simulink model "twolevelwithconstantdcvoltage_tuned_2017"  (R2017b)
settings: Solver=FixedStepAuto  StartTime=0.0  StopTime=30  FixedStep=Ts  MaxStep=1e-4  RelTol=1e-3  EnableMultiTasking=on
undefined symbols (not defined in the file): Ts
libraries: powerlib x18, powerlib_meascontrol x10, simulink x3
settings Model: Creator=Eren  LastModifiedBy=Eren
settings DataIOCC: LimitDataPoints=on
settings OptimizationCC: LifeSpan=inf
settings DebuggingCC: AllowSymbolicDim=off  SFUnexpectedBacktrackingDiag=warning  SFNoUnconditionalDefaultTransitionDiag=warning  SFExecutionAtInitializationDiag=none
settings ModelReferenceCC: PropagateSignalLabelsOutOfModel=off
settings CodeAppCC: StateflowObjectComments=on
settings GRTTargetCC: TargetLangStandard=C89/C90 (ANSI)
settings ConfigComp: CovMetricSettings=dw  CovHtmlReporting=on  CovSaveCumulativeToWorkspaceVar=on  CovSaveSingleToWorkspaceVar=on  CovExternalEMLEnable=off
settings SimscapeCC: SimscapeNormalizeSystem=off

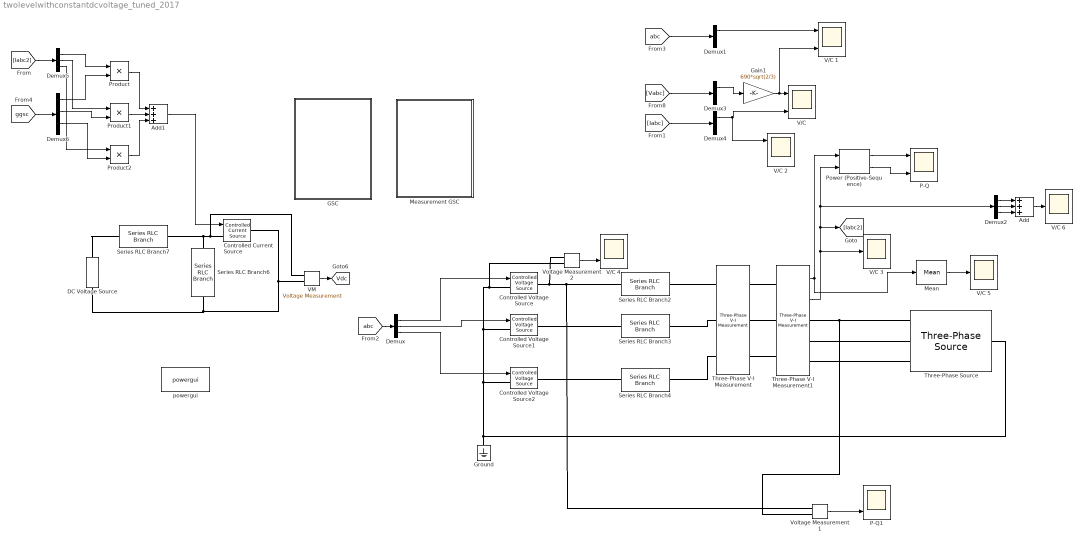
== system twolevelwithconstantdcvoltage_tuned_2017 ==
  Add : Sum  Inputs=3
  Add1 : Sum  Inputs=3
  Controlled Current Source : powerlib/Electrical Sources/Controlled Current Source  Initialize=off  Source_Type=AC  Amplitude=0  Phase=0  Frequency=0  Measurements=None
  Controlled Voltage Source : powerlib/Electrical Sources/Controlled Voltage Source  Initialize=off  Source_Type=AC  Amplitude=0  Phase=0  Frequency=0  Measurements=None
  Controlled Voltage Source1 : powerlib/Electrical Sources/Controlled Voltage Source  Initialize=on  Source_Type=AC  Amplitude=0  Phase=0  Frequency=0  Measurements=None
  Controlled Voltage Source2 : powerlib/Electrical Sources/Controlled Voltage Source  Initialize=on  Source_Type=AC  Amplitude=0  Phase=0  Frequency=0  Measurements=None
  DC Voltage Source : powerlib/Electrical Sources/DC Voltage Source  Amplitude=1300  Measurements=None
  Demux{,1..5} (6 alike) : Demux  Outputs=3
  Demux6 : Demux  Outputs=6
  GSC : Subsystem
  Gain1 : Gain  Gain=690*sqrt(2/3)
  Ground : powerlib/Elements/Ground  LConnTagsString=a
  Mean : powerlib_meascontrol/Measurements/Mean  Freq=50  Vinit=0  Ts=Ts
  Measurement GSC : Subsystem
  P-Q : Scope  NumInputPorts=2
  P-Q1 : Scope  NumInputPorts=2
  Power (Positive-Sequence) : powerlib_meascontrol/Measurements/Power (Positive-Sequence)  Freq=50  Vinit=[0, 0]  Iinit=[0, 0]  Ts=Ts
      settings: SourceProductName=Simscape Power Systems  SourceProductBaseCode=PS
  Product : Product
  Product1 : Product
  Product2 : Product
  Series RLC Branch2 : powerlib/Elements/Series RLC Branch  LConnTagsString=__new0  RConnTagsString=__new0  BranchType=L  Resistance=1  Inductance=2e-4  SetiL0=off  InitialCurrent=0  Capacitance=1e-6  Setx0=off  InitialVoltage=0  Measurements=None
  Series RLC Branch3 : powerlib/Elements/Series RLC Branch  LConnTagsString=__new0  RConnTagsString=__new0  BranchType=L  Resistance=1  Inductance=2e-4  SetiL0=off  InitialCurrent=0  Capacitance=1e-6  Setx0=off  InitialVoltage=0  Measurements=None
  Series RLC Branch4 : powerlib/Elements/Series RLC Branch  LConnTagsString=__new0  RConnTagsString=__new0  BranchType=L  Resistance=1  Inductance=2e-4  SetiL0=off  InitialCurrent=0  Capacitance=1e-6  Setx0=off  InitialVoltage=0  Measurements=None
  Series RLC Branch6 : powerlib/Elements/Series RLC Branch  LConnTagsString=__new0  RConnTagsString=__new0  BranchType=C  Resistance=1  Inductance=1e-4  SetiL0=off  InitialCurrent=0  Capacitance=27e-3  Setx0=off  InitialVoltage=0  Measurements=None
  Series RLC Branch7 : powerlib/Elements/Series RLC Branch  LConnTagsString=__new0  RConnTagsString=__new0  BranchType=R  Resistance=(120000)/(2.75*10^6)  Inductance=1e-3  SetiL0=off  InitialCurrent=0  Capacitance=1e-6  Setx0=off  InitialVoltage=0  Measurements=None
  Three-Phase V-I Measurement : powerlib/Measurements/Three-Phase V-I Measurement  VoltageMeasurement=phase-to-ground  SetLabelV=on  LabelV=Vabc  Vpu=on  VpuLL=off  CurrentMeasurement=yes  SetLabelI=on  LabelI=Iabc  Ipu=on  Pbase=2.75e6  Vbase=690  OutputType=Complex  PhasorSimulation=off  PSBequivalent=0
  Three-Phase V-I Measurement1 : powerlib/Measurements/Three-Phase V-I Measurement  VoltageMeasurement=phase-to-ground  SetLabelV=off  LabelV=Vabc  Vpu=off  VpuLL=off  CurrentMeasurement=yes  SetLabelI=off  LabelI=Iabc  Ipu=off  Pbase=2.75e6  Vbase=690  OutputType=Complex  PhasorSimulation=off  PSBequivalent=0
  Three-Phase Source : powerlib/Electrical Sources/Three-Phase Source  InternalConnection=Yn  VoltagePhases=off  Voltage=690  PhaseAngle=0  Voltage_phases=[25e3 25e3 25e3]/sqrt(3)  PhaseAngles_phases=[0 -120 +120]  Frequency=50  NonIdealSource=on  SpecifyImpedance=off  Resistance=3e-5  Inductance=1e-5  ShortCircuitLevel=500e6  BaseVoltage=690  XRratio=7  BusType=swing  Pref=10e3  Qref=0  Prefabc=[10e3, 10e3, 10e3]  Qrefabc=[0, 0, 0]  Qmin=-inf  Qmax=inf
  V/C {,1..2,4} (4 alike) : Scope  NumInputPorts=2
  V/C 3 : Scope
  V/C 5 : Scope
  V/C 6 : Scope
  VM : powerlib/Measurements/Voltage Measurement  PhasorSimulation=off  OutputType=Complex  PSBequivalent=0
  Voltage Measurement1 : powerlib/Measurements/Voltage Measurement  PhasorSimulation=off  OutputType=Complex  PSBequivalent=0
  Voltage Measurement2 : powerlib/Measurements/Voltage Measurement  PhasorSimulation=off  OutputType=Complex  PSBequivalent=0
  powergui : powerlib/powergui  Priority=1  SimulationMode=Continuous  SampleTime=50e-6  frequency=60  Iterations=50  frequencyindice=60  Pbase=100e6  ErrMax=1e-4  UnitsV=kV  UnitsW=MW  buscounter=0  FunctionMessages=off  echomessages=off  EnableUseOfTLC=off  CurrentSourceSwitches=off  DisableSnubberDevices=off  DisableRonSwitches=off  DisableVfSwitches=off  DisplayEquations=off  SolverType=Tustin/Backward Euler (TBE)  Interpol=off  ExternalGateDelay=off  methode=off  Ts=100  x0status=blocks  SPID=on  SwTol=0  HookPort=off  RestoreLinks=warning  ResistiveCurrentMeasurement=off  Frange=[0:2:500]  Ylog=off  Xlog=on  ShowGrid=off  save=off  variable=ZData  structure=0  ZoomFFT=off  StartTime=0.0  cycles=1  DisplayStyle=1  fundamental=60  FreqAxis=off  MaxFrequency=1000  frequencyindicesteady=1  RmsSteady=1  display=off
  tag scope: Vdc=global
  wires:
  Demux4/1 -> V/C 2/1, "V/C "/2
  Demux3/1 -> Gain1/1
  [Vabc] -> Demux3/1
  VM/1 -> [Vdc]
  Power (Positive-Sequence)/1 -> P-Q/1
  Power (Positive-Sequence)/2 -> P-Q/2
  [Iabc] -> Demux4/1
  Three-Phase V-I Measurement1/1 -> Power (Positive-Sequence)/1, Mean/1
  Three-Phase V-I Measurement1/2 -> V/C 3/1, [Iabc2], Power (Positive-Sequence)/2, Demux2/1
  [abc] -> Demux/1
  Demux/1 -> Controlled Voltage Source/1
  Demux/2 -> Controlled Voltage Source1/1
  Demux/3 -> Controlled Voltage Source2/1
  [abc] -> Demux1/1
  Demux1/1 -> V/C 1/1
  Gain1/1 -> V/C 1/2, "V/C "/1
  Voltage Measurement1/1 -> P-Q1/2
  Voltage Measurement2/1 -> V/C 4/2
  Mean/1 -> V/C 5/1
  Demux2/1 -> Add/1
  Demux2/2 -> Add/2
  Demux2/3 -> Add/3
  Add/1 -> V/C 6/1
  [Iabc2] -> Demux5/1
  [ggsc] -> Demux6/1
  Demux5/1 -> Product/1
  Demux6/1 -> Product/2
  Demux5/2 -> Product1/1
  Demux6/3 -> Product1/2
  Demux5/3 -> Product2/1
  Demux6/5 -> Product2/2
  Product/1 -> Add1/1
  Product1/1 -> Add1/2
  Product2/1 -> Add1/3
  Add1/1 -> Controlled Current Source/1
  connections:
  Three-Phase V-I Measurement1/RConn1 -- Three-Phase Source/RConn1 -- Voltage Measurement1/LConn2
  Series RLC Branch7/LConn1 -- DC Voltage Source/RConn1
  Series RLC Branch2/RConn1 -- Three-Phase V-I Measurement/LConn1
  Series RLC Branch6/RConn1 -- VM/LConn2 -- Controlled Current Source/RConn1 -- DC Voltage Source/LConn1
  Three-Phase V-I Measurement/RConn1 -- Three-Phase V-I Measurement1/LConn1
  Three-Phase V-I Measurement1/LConn2 -- Three-Phase V-I Measurement/RConn2
  Three-Phase V-I Measurement/RConn3 -- Three-Phase V-I Measurement1/LConn3
  Controlled Voltage Source/LConn1 -- Voltage Measurement2/LConn2 -- Ground/LConn1 -- Three-Phase Source/LConn1 -- Controlled Voltage Source2/LConn1 -- Controlled Voltage Source1/LConn1
  Series RLC Branch3/LConn1 -- Controlled Voltage Source1/RConn1
  Series RLC Branch4/RConn1 -- Three-Phase V-I Measurement/LConn3
  Series RLC Branch2/LConn1 -- Voltage Measurement1/LConn1 -- Voltage Measurement2/LConn1 -- Controlled Voltage Source/RConn1
  Series RLC Branch3/RConn1 -- Three-Phase V-I Measurement/LConn2
  Series RLC Branch4/LConn1 -- Controlled Voltage Source2/RConn1
  Three-Phase Source/RConn2 -- Three-Phase V-I Measurement1/RConn2
  Three-Phase Source/RConn3 -- Three-Phase V-I Measurement1/RConn3
  Series RLC Branch6/LConn1 -- VM/LConn1 -- Controlled Current Source/LConn1 -- Series RLC Branch7/RConn1

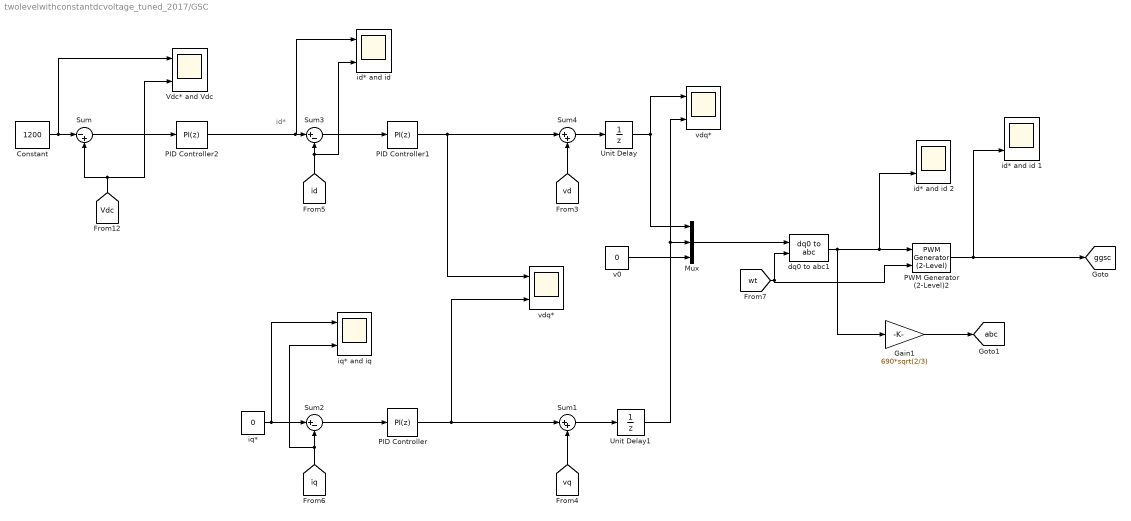
== system twolevelwithconstantdcvoltage_tuned_2017/GSC ==
  note: id*
  Constant : Constant  Value=1200
  Gain1 : Gain  Gain=690*sqrt(2/3)
  Mux : Mux  Inputs=3
  PID Controller : simulink/Continuous/PID Controller  Controller=PI  TimeDomain=Discrete-time  SampleTime=-1  IntegratorMethod=Forward Euler  FilterMethod=Forward Euler  Form=Parallel  UseFilter=on  ControllerParametersSource=internal  P=49.7840114924255  I=37375.3273073798  D=0  N=100  InitialConditionSource=internal  InitialConditionForIntegrator=0  InitialConditionForFilter=0  ExternalReset=none  LimitOutput=on  UpperSaturationLimit=2  LowerSaturationLimit=-2  LinearizeAsGain=on  AntiWindupMode=none  Kb=1  TrackingMode=off  Kt=1  PParamMin=[]  PParamMax=[]  IParamMin=[]  IParamMax=[]  DParamMin=[]  DParamMax=[]  NParamMin=[]  NParamMax=[]  KbParamMin=[]  KbParamMax=[]  KtParamMin=[]  KtParamMax=[]  POutMin=[]  POutMax=[]  IOutMin=[]  IOutMax=[]  DOutMin=[]  DOutMax=[]  NOutMin=[]  NOutMax=[]  KbOutMin=[]  KbOutMax=[]  KtOutMin=[]  KtOutMax=[]  IntegratorOutMin=[]  IntegratorOutMax=[]  FilterOutMin=[]  FilterOutMax=[]  SumOutMin=[]  SumOutMax=[]  SumI1OutMin=[]  SumI1OutMax=[]  SumI2OutMin=[]  SumI2OutMax=[]  SumI3OutMin=[]  SumI3OutMax=[]  SumDOutMin=[]  SumDOutMax=[]  SaturationOutMin=[]  SaturationOutMax=[]  IntegratorContinuousStateAttributes=''  IntegratorStateMustResolveToSignalObject=off  IntegratorRTWStateStorageClass=Auto  FilterContinuousStateAttributes=''  FilterStateMustResolveToSignalObject=off  FilterRTWStateStorageClass=Auto  DifferentiatorICPrevScaledInput=0  DifferentiatorOutMin=[]  DifferentiatorOutMax=[]  InitialConditionSetting=State (most efficient)  FilterDiffOutCoefMin=[]  FilterDiffOutCoefMax=[]  SumDenOutMin=[]  SumDenOutMax=[]  SumNumOutMin=[]  SumNumOutMax=[]  ReciprocalOutMin=[]  ReciprocalOutMax=[]  DivideOutMin=[]  DivideOutMax=[]  TunerSelectOption=Transfer Function Based (PID Tuner App)
  PID Controller1 : simulink/Continuous/PID Controller  Controller=PI  TimeDomain=Discrete-time  SampleTime=-1  IntegratorMethod=Forward Euler  FilterMethod=Forward Euler  Form=Parallel  UseFilter=on  ControllerParametersSource=internal  P=34.0158922210728  I=17493.3134828869  D=0  N=100  InitialConditionSource=internal  InitialConditionForIntegrator=0  InitialConditionForFilter=0  ExternalReset=none  LimitOutput=on  UpperSaturationLimit=1  LowerSaturationLimit=-1  LinearizeAsGain=on  AntiWindupMode=none  Kb=1  TrackingMode=off  Kt=1  PParamMin=[]  PParamMax=[]  IParamMin=[]  IParamMax=[]  DParamMin=[]  DParamMax=[]  NParamMin=[]  NParamMax=[]  KbParamMin=[]  KbParamMax=[]  KtParamMin=[]  KtParamMax=[]  POutMin=[]  POutMax=[]  IOutMin=[]  IOutMax=[]  DOutMin=[]  DOutMax=[]  NOutMin=[]  NOutMax=[]  KbOutMin=[]  KbOutMax=[]  KtOutMin=[]  KtOutMax=[]  IntegratorOutMin=[]  IntegratorOutMax=[]  FilterOutMin=[]  FilterOutMax=[]  SumOutMin=[]  SumOutMax=[]  SumI1OutMin=[]  SumI1OutMax=[]  SumI2OutMin=[]  SumI2OutMax=[]  SumI3OutMin=[]  SumI3OutMax=[]  SumDOutMin=[]  SumDOutMax=[]  SaturationOutMin=[]  SaturationOutMax=[]  IntegratorContinuousStateAttributes=''  IntegratorStateMustResolveToSignalObject=off  IntegratorRTWStateStorageClass=Auto  FilterContinuousStateAttributes=''  FilterStateMustResolveToSignalObject=off  FilterRTWStateStorageClass=Auto  DifferentiatorICPrevScaledInput=0  DifferentiatorOutMin=[]  DifferentiatorOutMax=[]  InitialConditionSetting=State (most efficient)  FilterDiffOutCoefMin=[]  FilterDiffOutCoefMax=[]  SumDenOutMin=[]  SumDenOutMax=[]  SumNumOutMin=[]  SumNumOutMax=[]  ReciprocalOutMin=[]  ReciprocalOutMax=[]  DivideOutMin=[]  DivideOutMax=[]  TunerSelectOption=Transfer Function Based (PID Tuner App)
  PID Controller2 : simulink/Continuous/PID Controller  Controller=PI  TimeDomain=Discrete-time  SampleTime=-1  IntegratorMethod=Forward Euler  FilterMethod=Forward Euler  Form=Parallel  UseFilter=on  ControllerParametersSource=internal  P=83655.09858372  I=42227.4588739829  D=0  N=100  InitialConditionSource=internal  InitialConditionForIntegrator=0  InitialConditionForFilter=0  ExternalReset=none  LimitOutput=off  UpperSaturationLimit=inf  LowerSaturationLimit=-inf  LinearizeAsGain=on  AntiWindupMode=none  Kb=1  TrackingMode=off  Kt=1  PParamMin=[]  PParamMax=[]  IParamMin=[]  IParamMax=[]  DParamMin=[]  DParamMax=[]  NParamMin=[]  NParamMax=[]  KbParamMin=[]  KbParamMax=[]  KtParamMin=[]  KtParamMax=[]  POutMin=[]  POutMax=[]  IOutMin=[]  IOutMax=[]  DOutMin=[]  DOutMax=[]  NOutMin=[]  NOutMax=[]  KbOutMin=[]  KbOutMax=[]  KtOutMin=[]  KtOutMax=[]  IntegratorOutMin=[]  IntegratorOutMax=[]  FilterOutMin=[]  FilterOutMax=[]  SumOutMin=[]  SumOutMax=[]  SumI1OutMin=[]  SumI1OutMax=[]  SumI2OutMin=[]  SumI2OutMax=[]  SumI3OutMin=[]  SumI3OutMax=[]  SumDOutMin=[]  SumDOutMax=[]  SaturationOutMin=[]  SaturationOutMax=[]  IntegratorContinuousStateAttributes=''  IntegratorStateMustResolveToSignalObject=off  IntegratorRTWStateStorageClass=Auto  FilterContinuousStateAttributes=''  FilterStateMustResolveToSignalObject=off  FilterRTWStateStorageClass=Auto  DifferentiatorICPrevScaledInput=0  DifferentiatorOutMin=[]  DifferentiatorOutMax=[]  InitialConditionSetting=State (most efficient)  FilterDiffOutCoefMin=[]  FilterDiffOutCoefMax=[]  SumDenOutMin=[]  SumDenOutMax=[]  SumNumOutMin=[]  SumNumOutMax=[]  ReciprocalOutMin=[]  ReciprocalOutMax=[]  DivideOutMin=[]  DivideOutMax=[]  TunerSelectOption=Transfer Function Based (PID Tuner App)
  PWM Generator (2-Level)2 : powerlib_meascontrol/Pulse & Signal Generators/PWM Generator (2-Level)  ModulatorType=Three-phase bridge (6 pulses)  ModulatorMode=Synchronized  Fc=50*60  Pc=90  nF=100  MinMax="[ -1  1 ]"  SamplingTechnique=Natural  ModulatingSignals=off  m=0.8  Freq=60  Phase=0  Ts=Ts  ShowCarrierOutport=off
      settings: SourceProductName=Simscape Power Systems
  Sum : Sum  Inputs=|-+
  Sum1 : Sum  Inputs=|++
  Sum2 : Sum  Inputs=|+-
  Sum3 : Sum  Inputs=|+-
  Sum4 : Sum  Inputs=|++
  Unit Delay : UnitDelay  SampleTime=Ts
  Unit Delay1 : UnitDelay  SampleTime=Ts
  Vdc* and Vdc : Scope  NumInputPorts=2
  dq0 to abc1 : powerlib_meascontrol/Transformations/dq0 to abc  Alignment=90 degrees behind phase A axis
  "id* and id " : Scope  NumInputPorts=2
  id* and id 1 : Scope  NumInputPorts=2
  id* and id 2 : Scope  NumInputPorts=2
  iq* : Constant  Value=0
  "iq* and iq " : Scope  NumInputPorts=2
  v0 : Constant  Value=0
  vdq* : Scope  NumInputPorts=2
  "vdq* " : Scope  NumInputPorts=2
  tag scope: abc=global, ggsc=global
  wires:
  PWM Generator (2-Level)2/1 -> id* and id 1/2, [ggsc]
  iq*/1 -> "iq* and iq "/1, Sum2/1
  Sum3/1 -> PID Controller1/1
  [iq] -> Sum2/2, "iq* and iq "/2
  PID Controller/1 -> Sum1/1, vdq*/2
  [vq] -> Sum1/2
  [id] -> "id* and id "/2, Sum3/2
  Sum2/1 -> PID Controller/1
  [vd] -> Sum4/2
  PID Controller1/1 -> Sum4/1, vdq*/1
  Sum4/1 -> Unit Delay/1
  Mux/1 -> dq0 to abc1/1
  [wt] -> dq0 to abc1/2, PWM Generator (2-Level)2/2
  Sum1/1 -> Unit Delay1/1
  v0/1 -> Mux/3
  [Vdc] -> Vdc* and Vdc/2, Sum/2
  Sum/1 -> PID Controller2/1
  Constant/1 -> Vdc* and Vdc/1, Sum/1
  PID Controller2/1 -> "id* and id "/1, Sum3/1
  dq0 to abc1/1 -> Gain1/1, id* and id 2/2, PWM Generator (2-Level)2/1
  Gain1/1 -> [abc]
  Unit Delay/1 -> Mux/1, "vdq* "/1
  Unit Delay1/1 -> "vdq* "/2, Mux/2

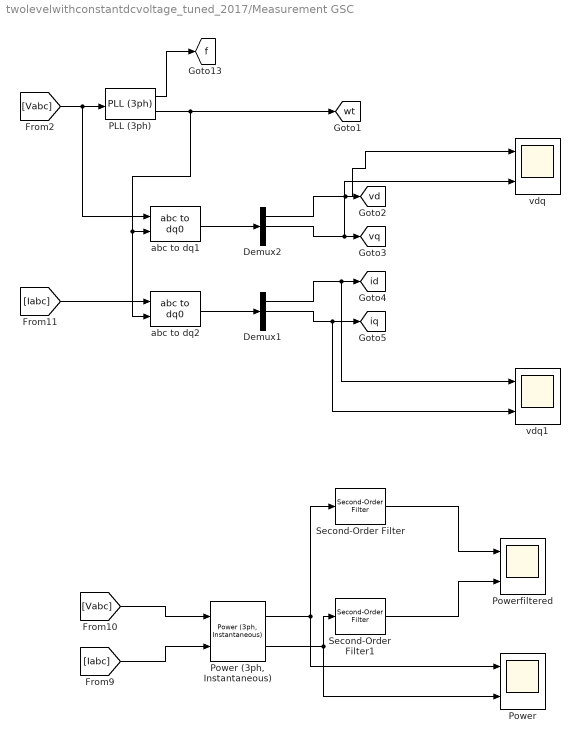
== system twolevelwithconstantdcvoltage_tuned_2017/Measurement GSC ==
  Demux1 : Demux  Outputs=3
  Demux2 : Demux  Outputs=3
  PLL (3ph) : powerlib_meascontrol/PLL/PLL (3ph)  Fmin=45  Par_Init=[0, 50]  ParK=[180, 3200, 1]  TcD=1e-4  MaxRateChangeFreq=12  FilterCutOffFreq=25  Ts=Ts  AGC=on
  Power : Scope  NumInputPorts=2
  "Power (3ph, Instantaneous)" : powerlib_meascontrol/Measurements/Power (3ph, Instantaneous)
      settings: SourceProductName=Simscape Power Systems
  "Powerfiltered " : Scope  NumInputPorts=2
  Second-Order Filter : powerlib_meascontrol/Filters/Second-Order Filter  FilterType=Lowpass  Fo=50  Zeta=0.707  Ts=Ts  Initialize=off  Vac_Init="[0,  0,  60]"  Vdc_Init=0  PlotResponse=off  FreqRange=[0, 500, 1]
      settings: SourceProductName=Simscape Power Systems  SourceProductBaseCode=PS
  Second-Order Filter1 : powerlib_meascontrol/Filters/Second-Order Filter  FilterType=Lowpass  Fo=100  Zeta=0.707  Ts=0  Initialize=off  Vac_Init="[0,  0,  60]"  Vdc_Init=0  PlotResponse=off  FreqRange=[0, 500, 1]
      settings: SourceProductName=Simscape Power Systems  SourceProductBaseCode=PS
  abc to dq1 : powerlib_meascontrol/Transformations/abc to dq0  Alignment=90 degrees behind phase A axis
  abc to dq2 : powerlib_meascontrol/Transformations/abc to dq0  Alignment=90 degrees behind phase A axis
  vdq : Scope  NumInputPorts=2
  vdq1 : Scope  NumInputPorts=2
  tag scope: f=global, id=global, iq=global, vd=global, vq=global, wt=global
  wires:
  PLL (3ph)/1 -> [f]
  [Vabc] -> abc to dq1/1, PLL (3ph)/1
  PLL (3ph)/2 -> abc to dq1/2, abc to dq2/2, [wt]
  [Iabc] -> abc to dq2/1
  Demux2/1 -> vdq/1, [vd]
  Demux2/2 -> vdq/2, [vq]
  Demux1/1 -> vdq1/1, [id]
  Demux1/2 -> vdq1/2, [iq]
  abc to dq1/1 -> Demux2/1
  abc to dq2/1 -> Demux1/1
  "Power (3ph, Instantaneous)"/1 -> Power/1, Second-Order Filter/1
  "Power (3ph, Instantaneous)"/2 -> Power/2, Second-Order Filter1/1
  Second-Order Filter1/1 -> "Powerfiltered "/2
  Second-Order Filter/1 -> "Powerfiltered "/1
  [Vabc] -> "Power (3ph, Instantaneous)"/1
  [Iabc] -> "Power (3ph, Instantaneous)"/2
